simulink model "All"  (R2022b)
settings: Solver=FixedStepAuto  StartTime=0.0  StopTime=5  FixedStep=0.1  RelTol=1e-3
model workspace (MAT data in the model file):
  Sig = Simulink.Signal
  Sig.DataType = 'auto'
  Sig.Dimensions = -1
  Sig.DimensionsMode = 'auto'
  Sig.Complexity = 'auto'
  Sig.SampleTime = -1
  Sig.SamplingMode = 'auto'
values from neighbouring files (symbols this model uses):
  Kt = 10    [testCase.m]
  Kx = 5    [testCase.m]
  NoisePower = 0.01    [testCase.m]
  SysQ = 0.01    [testCase.m]
  timeStep = 0.1    [testCase.m]
libraries: simulink_extras x4, sharedTrackingLibrary x1, simulink x1
settings Model: Creator=The MathWorks, Inc.  LastModifiedBy=MuAyman
settings SolverCC: AlgebraicLoopSolver=TrustRegion
settings DebuggingCC: UnconnectedInputMsg=warning  UnconnectedOutputMsg=warning  UnconnectedLineMsg=warning  SymbolicDimsDataTypeCodeGenerationDiagnostic=none  SFMachineParentedDataDiag=warning
settings ModelReferenceCC: EnableRefExpFcnMdlSchedulingChecks=on
settings RTWCC: DLArmComputeVersion=19.05

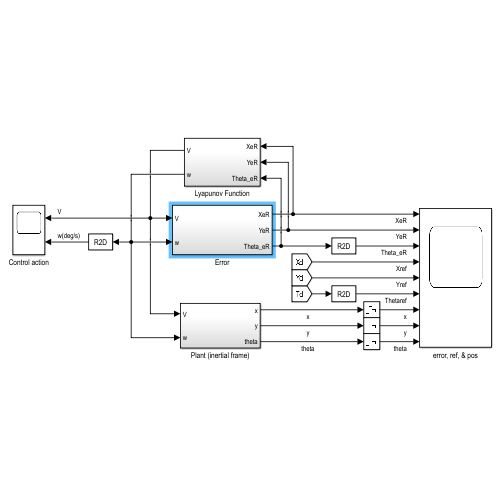
[thumbnail: Simulink's stored preview of the top-level diagram]
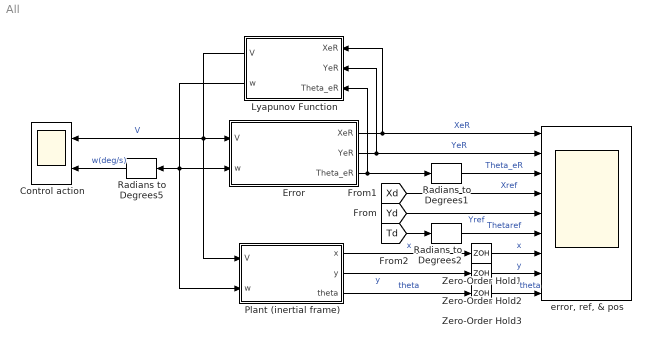
== system All ==
  Control action : Scope  NumInputPorts=2
  Error : Subsystem
  Lyapunov Function : Subsystem
  Plant (inertial frame) : Subsystem
  Radians to Degrees1 : simulink_extras/Transformations/Radians to Degrees
  Radians to Degrees2 : simulink_extras/Transformations/Radians to Degrees
  Radians to Degrees5 : simulink_extras/Transformations/Radians to Degrees
  Zero-Order Hold1 : ZeroOrderHold  SampleTime=timeStep
  Zero-Order Hold2 : ZeroOrderHold  SampleTime=timeStep
  Zero-Order Hold3 : ZeroOrderHold  SampleTime=timeStep
  "error, ref, & pos" : Scope  NumInputPorts=9
  wires:
  Radians to Degrees5/1 -> Control action/2  "w(deg/s)"
  Error/2(YeR) -> Lyapunov Function/2(YeR), "error, ref, & pos"/2  "YeR"
  Error/3(Theta_eR) -> Lyapunov Function/3(Theta_eR), Radians to Degrees1/1
  Error/1(XeR) -> Lyapunov Function/1(XeR), "error, ref, & pos"/1  "XeR"
  Radians to Degrees1/1 -> "error, ref, & pos"/3  "Theta_eR"
  [Xd] -> "error, ref, & pos"/4  "Xref"
  [Yd] -> "error, ref, & pos"/5  "Yref"
  [Td] -> Radians to Degrees2/1
  Lyapunov Function/2(w) -> Error/2(w), Radians to Degrees5/1, Plant (inertial frame)/2(w)
  Plant (inertial frame)/3(theta) -> Zero-Order Hold3/1  "theta"
  Lyapunov Function/1(V) -> Control action/1, Plant (inertial frame)/1(V), Error/1(V)  "V"
  Plant (inertial frame)/2(y) -> Zero-Order Hold2/1  "y"
  Plant (inertial frame)/1(x) -> Zero-Order Hold1/1  "x"
  Radians to Degrees2/1 -> "error, ref, & pos"/6  "Thetaref"
  Zero-Order Hold1/1 -> "error, ref, & pos"/7  "x"
  Zero-Order Hold2/1 -> "error, ref, & pos"/8  "y"
  Zero-Order Hold3/1 -> "error, ref, & pos"/9  "theta"

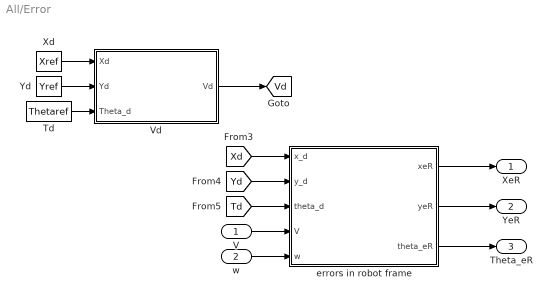
== system All/Error ==
  V : Inport
  w : Inport  Port=2
  Td : FromWorkspace  VariableName=Thetaref  SampleTime=timeStep  OutputAfterFinalValue=Holding final value
  Vd : Subsystem
  Xd : FromWorkspace  VariableName=Xref  SampleTime=timeStep  OutputAfterFinalValue=Holding final value
  Yd : FromWorkspace  VariableName=Yref  SampleTime=timeStep  OutputAfterFinalValue=Holding final value
  errors in robot frame : Subsystem
  XeR : Outport
  YeR : Outport  Port=2
  Theta_eR : Outport  Port=3
  tag scope: Vd=global
  wires:
  w/1 -> errors in robot frame/5(w)
  V/1 -> errors in robot frame/4(V)
  Vd/1(Vd) -> [Vd]
  Xd/1 -> Vd/1(Xd)
  Yd/1 -> Vd/2(Yd)
  errors in robot frame/2(yeR) -> YeR/1
  errors in robot frame/3(theta_eR) -> Theta_eR/1
  errors in robot frame/1(xeR) -> XeR/1
  [Yd] -> errors in robot frame/2(y_d)
  [Xd] -> errors in robot frame/1(x_d)
  [Td] -> errors in robot frame/3(theta_d)
  Td/1 -> Vd/3(Theta_d)

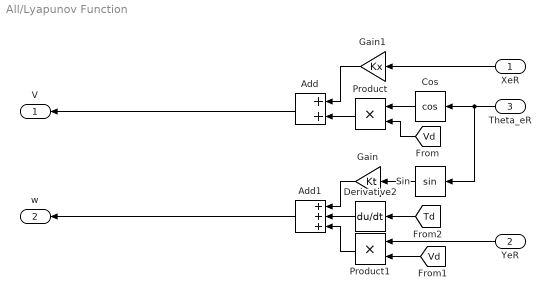
== system All/Lyapunov Function ==
  XeR : Inport
  YeR : Inport  Port=2
  Theta_eR : Inport  Port=3
  Add : Sum
  Add1 : Sum  Inputs=+++
  Cos : Trigonometry  Operator=cos
  Derivative2 : Derivative
  Gain : Gain  Gain=Kt
  Gain1 : Gain  Gain=Kx
  Product : Product
  Product1 : Product
  Sin : Trigonometry
  V : Outport
  w : Outport  Port=2
  wires:
  [Vd] -> Product1/2
  [Vd] -> Product/2
  Product/1 -> Add/2
  Sin/1 -> Gain/1
  [Td] -> Derivative2/1
  Cos/1 -> Product/1
  Gain1/1 -> Add/1
  Gain/1 -> Add1/1
  Product1/1 -> Add1/3
  XeR/1 -> Gain1/1
  Theta_eR/1 -> Sin/1, Cos/1
  Add1/1 -> w/1
  YeR/1 -> Product1/1
  Add/1 -> V/1
  Derivative2/1 -> Add1/2

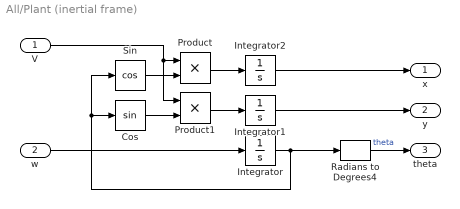
== system All/Plant (inertial frame) ==
  V : Inport
  w : Inport  Port=2
  Cos : Trigonometry
  Integrator : Integrator
  Integrator1 : Integrator
  Integrator2 : Integrator
  Product : Product
  Product1 : Product
  Radians to Degrees4 : simulink_extras/Transformations/Radians to Degrees
  Sin : Trigonometry  Operator=cos
  x : Outport
  y : Outport  Port=2
  theta : Outport  Port=3
  wires:
  Integrator/1 -> Cos/1, Sin/1, Radians to Degrees4/1
  w/1 -> Integrator/1
  Sin/1 -> Product/2
  Cos/1 -> Product1/2
  Product1/1 -> Integrator1/1
  Product/1 -> Integrator2/1
  Integrator1/1 -> y/1
  Integrator2/1 -> x/1
  V/1 -> Product1/1, Product/1
  Radians to Degrees4/1 -> theta/1  "theta"

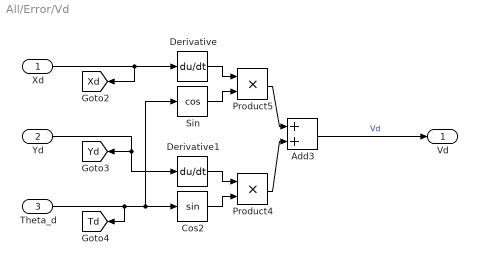
== system All/Error/Vd ==
  Xd : Inport
  Yd : Inport  Port=2
  Theta_d : Inport  Port=3
  Add3 : Sum
  Cos2 : Trigonometry
  Derivative : Derivative
  Derivative1 : Derivative
  Product4 : Product
  Product5 : Product
  Sin : Trigonometry  Operator=cos
  Vd : Outport
  tag scope: Td=global, Xd=global, Yd=global
  wires:
  Theta_d/1 -> [Td], Sin/1, Cos2/1
  Sin/1 -> Product5/2
  Derivative/1 -> Product5/1
  Product5/1 -> Add3/1
  Product4/1 -> Add3/2
  Cos2/1 -> Product4/2
  Derivative1/1 -> Product4/1
  Add3/1 -> Vd/1  "Vd"
  Yd/1 -> [Yd], Derivative1/1
  Xd/1 -> [Xd], Derivative/1

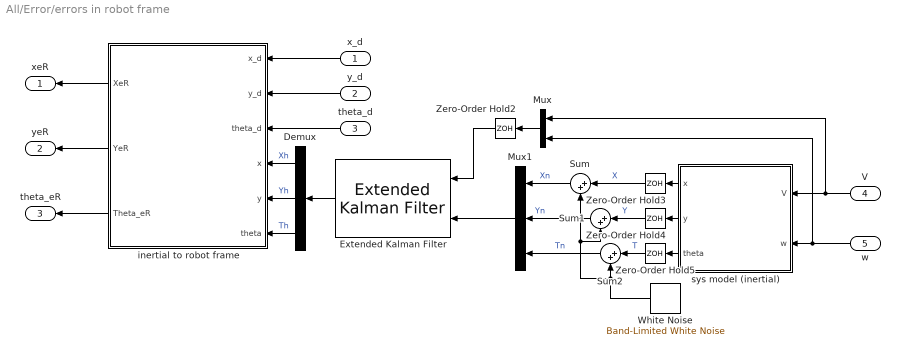
== system All/Error/errors in robot frame ==
  x_d : Inport
  y_d : Inport  Port=2
  theta_d : Inport  Port=3
  V : Inport  Port=4
  w : Inport  Port=5
  Demux : Demux  Outputs=3
  Extended Kalman Filter : sharedTrackingLibrary/Extended Kalman Filter  StateTransitionFcn=myRoboStateFun  HasStateTransitionJacobianFcn=off  StateTransitionJacobianFcn=A  HasAdditiveProcessNoise=Additive  ProcessNoise=SysQ*eye(3)  HasTimeVaryingProcessNoise=off  HasStateTransitionFcnExtraArgument=1  InitialState=startPos  InitialStateCovariance=1  MeasurementFcn1=myRoboOutputFun  HasMeasurementJacobianFcn1=off  MeasurementJacobianFcn1=C  HasMeasurementEnablePort1=off  HasAdditiveMeasurementNoise1=Additive  MeasurementNoise1=NoisePower*eye(3)  HasTimeVaryingMeasurementNoise1=off  HasMeasurementFcnExtraArgument1=0  HasMeasurementWrapping1=off  MeasurementFcn2=myMeasurementFcn  HasMeasurementJacobianFcn2=off  HasMeasurementEnablePort2=off  HasAdditiveMeasurementNoise2=Additive  MeasurementNoise2=1  HasTimeVaryingMeasurementNoise2=off  HasMeasurementFcnExtraArgument2=0  HasMeasurementWrapping2=off  MeasurementFcn3=myMeasurementFcn  HasMeasurementJacobianFcn3=off  HasMeasurementEnablePort3=off  HasAdditiveMeasurementNoise3=Additive  MeasurementNoise3=1  HasTimeVaryingMeasurementNoise3=off  HasMeasurementFcnExtraArgument3=0  HasMeasurementWrapping3=off  MeasurementFcn4=myMeasurementFcn  HasMeasurementJacobianFcn4=off  HasMeasurementEnablePort4=off  HasAdditiveMeasurementNoise4=Additive  MeasurementNoise4=1  HasTimeVaryingMeasurementNoise4=off  HasMeasurementFcnExtraArgument4=0  HasMeasurementWrapping4=off  MeasurementFcn5=myMeasurementFcn  HasMeasurementJacobianFcn5=off  HasMeasurementEnablePort5=off  HasAdditiveMeasurementNoise5=Additive  MeasurementNoise5=1  HasTimeVaryingMeasurementNoise5=off  HasMeasurementFcnExtraArgument5=0  HasMeasurementWrapping5=off  EnableMultirate=off  StateTransitionFcnSampleTime=1  MeasurementFcn1SampleTime=1  MeasurementFcn2SampleTime=1  MeasurementFcn3SampleTime=1  MeasurementFcn4SampleTime=1  MeasurementFcn5SampleTime=1  UseCurrentEstimator=on  OutputStateCovariance=off  DataType=double  SampleTime=timeStep  NumberOfMeasurements=1
  Mux : Mux  Inputs=2
  Mux1 : Mux  Inputs=3
  Sum : Sum  Inputs=|++
  Sum1 : Sum  Inputs=|++
  Sum2 : Sum  Inputs=|++
  White Noise : simulink/Sources/Band-Limited White Noise  Cov=NoisePower  Ts=timeStep  seed=[23341]
  Zero-Order Hold{2..5} (4 alike) : ZeroOrderHold  SampleTime=timeStep
  inertial to robot frame : Subsystem
  sys model (inertial) : Subsystem
  xeR : Outport
  yeR : Outport  Port=2
  theta_eR : Outport  Port=3
  wires:
  x_d/1 -> inertial to robot frame/1(x_d)
  y_d/1 -> inertial to robot frame/2(y_d)
  theta_d/1 -> inertial to robot frame/3(theta_d)
  inertial to robot frame/1(XeR) -> xeR/1
  inertial to robot frame/2(YeR) -> yeR/1
  inertial to robot frame/3(Theta_eR) -> theta_eR/1
  w/1 -> Mux/2, sys model (inertial)/2(w)
  V/1 -> Mux/1, sys model (inertial)/1(V)
  White Noise/1 -> Sum2/2, Sum1/2, Sum/2
  Sum/1 -> Mux1/1  "Xn"
  sys model (inertial)/1(x) -> Zero-Order Hold3/1
  sys model (inertial)/2(y) -> Zero-Order Hold4/1
  Sum1/1 -> Mux1/2  "Yn"
  sys model (inertial)/3(theta) -> Zero-Order Hold5/1
  Sum2/1 -> Mux1/3  "Tn"
  Mux/1 -> Zero-Order Hold2/1
  Mux1/1 -> Extended Kalman Filter/2
  Zero-Order Hold2/1 -> Extended Kalman Filter/1
  Zero-Order Hold3/1 -> Sum/1  "X"
  Zero-Order Hold4/1 -> Sum1/1  "Y"
  Zero-Order Hold5/1 -> Sum2/1  "T"
  Extended Kalman Filter/1 -> Demux/1
  Demux/1 -> inertial to robot frame/4(x)  "Xh"
  Demux/2 -> inertial to robot frame/5(y)  "Yh"
  Demux/3 -> inertial to robot frame/6(theta)  "Th"

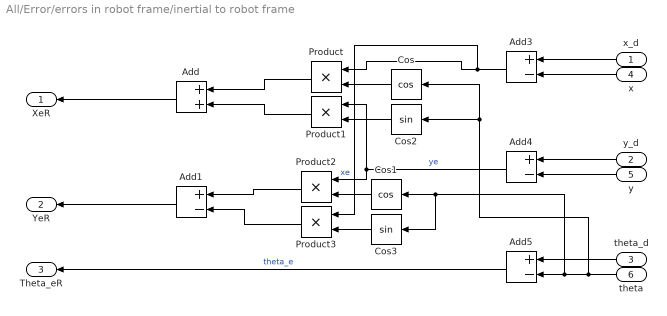
== system All/Error/errors in robot frame/inertial to robot frame ==
  x_d : Inport
  y_d : Inport  Port=2
  theta_d : Inport  Port=3
  x : Inport  Port=4
  y : Inport  Port=5
  theta : Inport  Port=6
  Add : Sum
  Add{1,3..5} (4 alike) : Sum  Inputs=+-
  Cos : Trigonometry  Operator=cos
  Cos1 : Trigonometry  Operator=cos
  Cos2 : Trigonometry
  Cos3 : Trigonometry
  Product{,1..3} (4 alike) : Product
  XeR : Outport
  YeR : Outport  Port=2
  Theta_eR : Outport  Port=3
  wires:
  theta_d/1 -> Add5/1
  Add4/1 -> Product2/1, Product1/1  "ye"
  y_d/1 -> Add4/1
  Add5/1 -> Theta_eR/1  "theta_e"
  x/1 -> Add3/2
  x_d/1 -> Add3/1
  y/1 -> Add4/2
  theta/1 -> Cos2/1, Cos/1, Cos3/1, Cos1/1, Add5/2
  Cos/1 -> Product/2
  Add3/1 -> Product3/1, Product/1  "xe"
  Product/1 -> Add/1
  Cos2/1 -> Product1/2
  Product1/1 -> Add/2
  Add/1 -> XeR/1
  Cos1/1 -> Product2/2
  Cos3/1 -> Product3/2
  Product2/1 -> Add1/1
  Product3/1 -> Add1/2
  Add1/1 -> YeR/1

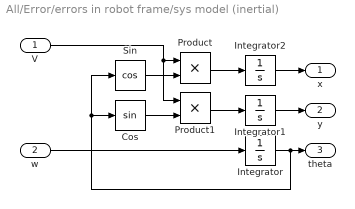
== system All/Error/errors in robot frame/sys model (inertial) ==
  V : Inport
  w : Inport  Port=2
  Cos : Trigonometry
  Integrator : Integrator
  Integrator1 : Integrator
  Integrator2 : Integrator
  Product : Product
  Product1 : Product
  Sin : Trigonometry  Operator=cos
  x : Outport
  y : Outport  Port=2
  theta : Outport  Port=3
  wires:
  Integrator/1 -> Cos/1, Sin/1, theta/1
  w/1 -> Integrator/1
  Sin/1 -> Product/2
  Cos/1 -> Product1/2
  Product1/1 -> Integrator1/1
  Product/1 -> Integrator2/1
  Integrator1/1 -> y/1
  Integrator2/1 -> x/1
  V/1 -> Product1/1, Product/1
